simulink model "Q11_simulink"  (R2020b)
settings: Solver=VariableStepAuto  StartTime=0.0  StopTime=200  RelTol=1e-3
settings Model: Creator=User  LastModifiedBy=User
settings SolverCC: AlgebraicLoopSolver=LineSearch

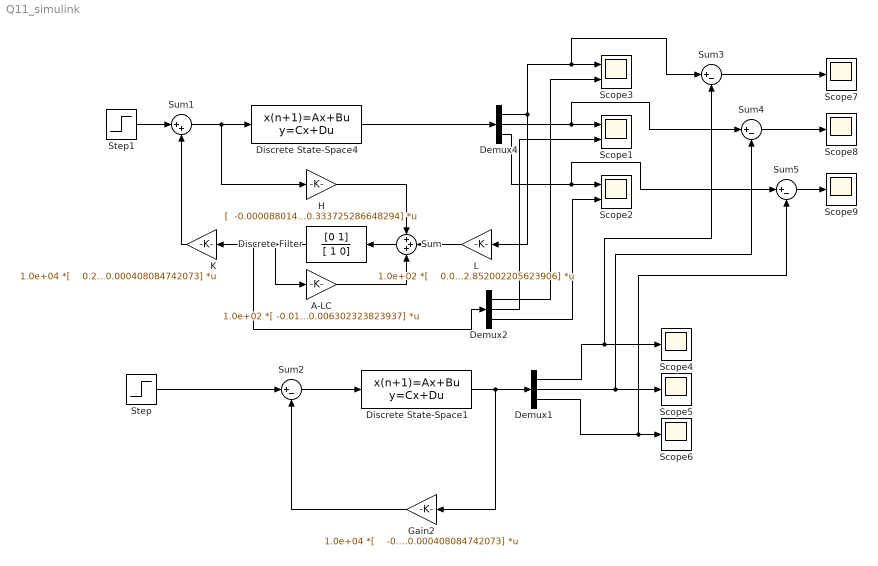
== system Q11_simulink ==
  A-LC : Gain  Gain=|  Multiplication=Matrix(K*u)
      | 1.0e+02 *[ -0.015127292849783  -0.211505575347728  -0.000006041895553
      |  ;  0.000737501490094   0.008824969025846   0.000000487045361
      | ;   2.852002205623906                   0   0.006302323823937]
  Demux1 : Demux  Outputs=3
  Demux2 : Demux  Outputs=3
  Demux4 : Demux  Outputs=3
  Discrete Filter : DiscreteFilter  Numerator=[0 1]  Denominator=[ 1 0]  SampleTime=5
  Discrete State-Space1 : DiscreteStateSpace  A=|  B=|  C=[1 0 0; 0 1 0 ; 0 0 1]  D=[0;0;0]  InitialCondition=10  SampleTime=5
      A=|
      | [ 1.000000000000000 -21.150557534772830  -0.000604189555321
      |          ;          0   0.882496902584595   0.000048704536076
      |           ;         0                   0   0.630232382393690]
      B=|
      | [  -0.000088014915701
      |  ;  0.000011188695469
      |  ;  0.333725286648294]
  Discrete State-Space4 : DiscreteStateSpace  A=|  B=|  C=[1 0 0; 0 1 0 ; 0 0 1]  D=[0;0;0]  InitialCondition=1  SampleTime=5
      A=|
      | [1.000000000000000 -21.150557534772830  -0.000604189555321
      |        ;            0   0.882496902584595   0.000048704536076
      |             ;       0                   0   0.630232382393690]
      B=|
      | [  -0.000088014915701
      |  ;  0.000011188695469
      |  ;  0.333725286648294]
  Gain2 : Gain  Gain=|  Multiplication=Matrix(K*u)
      | 1.0e+04 *[
      | 
      |    -0.217959452645970  8.571244823702385  0.000408084742073]
  H : Gain  Gain=|  Multiplication=Matrix(K*u)
      | [  -0.000088014915701
      |  ;  0.000011188695469
      |   ; 0.333725286648294]
  K : Gain  Gain=|  Multiplication=Matrix(K*u)
      | 1.0e+04 *[
      | 
      |    0.217959452645970  -8.571244823702385  -0.000408084742073]
  L : Gain  Gain=|  Multiplication=Matrix(K*u)
      | 1.0e+02 *[
      | 
      |    0.025127292849783
      |   -0.000737501490094
      |   -2.852002205623906]
  Scope1 : Scope  NumInputPorts=2
  Scope2 : Scope  NumInputPorts=2
  Scope3 : Scope  NumInputPorts=2
  Scope{4..9} (6 alike) : Scope
  Step : Step  Time=0  SampleTime=0
  Step1 : Step  Time=0  SampleTime=0
  Sum : Sum  Inputs=+++
  Sum1 : Sum  Inputs=|++
  Sum{2..5} (4 alike) : Sum  Inputs=|+-
  wires:
  Demux2/3 -> Scope2/2
  Demux2/2 -> Scope1/2
  Demux2/1 -> Scope3/2
  Sum/1 -> Discrete Filter/1
  Sum1/1 -> H/1, Discrete State-Space4/1
  Demux4/2 -> Sum4/1, Scope1/1
  Step1/1 -> Sum1/1
  Demux4/1 -> Sum3/1, Scope3/1, L/1
  K/1 -> Sum1/2
  Demux4/3 -> Sum5/1, Scope2/1
  Discrete State-Space4/1 -> Demux4/1
  L/1 -> Sum/2
  A-LC/1 -> Sum/3
  H/1 -> Sum/1
  Discrete Filter/1 -> A-LC/1, K/1, Demux2/1
  Step/1 -> Sum2/1
  Sum2/1 -> Discrete State-Space1/1
  Demux1/2 -> Sum4/2, Scope5/1
  Gain2/1 -> Sum2/2
  Discrete State-Space1/1 -> Gain2/1, Demux1/1
  Demux1/3 -> Sum5/2, Scope6/1
  Demux1/1 -> Sum3/2, Scope4/1
  Sum4/1 -> Scope8/1
  Sum3/1 -> Scope7/1
  Sum5/1 -> Scope9/1
